simulink model "single_phase_trans_short_circ_test"  (R2024b)
settings: Solver=VariableStepAuto  StartTime=0.0  StopTime=1  RelTol=1e-3
libraries: spsRMSLib x2, spsACVoltageSourceLib x1, spsCurrentMeasurementLib x1, spsLinearTransformerLib x1, eePowerMeasurement x1, spsVoltageMeasurementLib x1, sps_lib x1
settings Model: Creator=msi-nb  LastModifiedBy=msi-nb

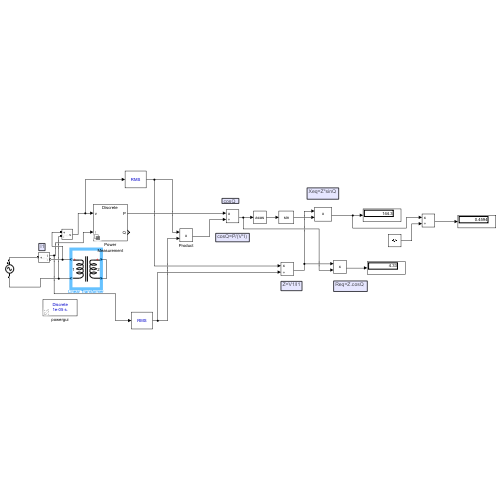
[thumbnail: Simulink's stored preview of the top-level diagram]
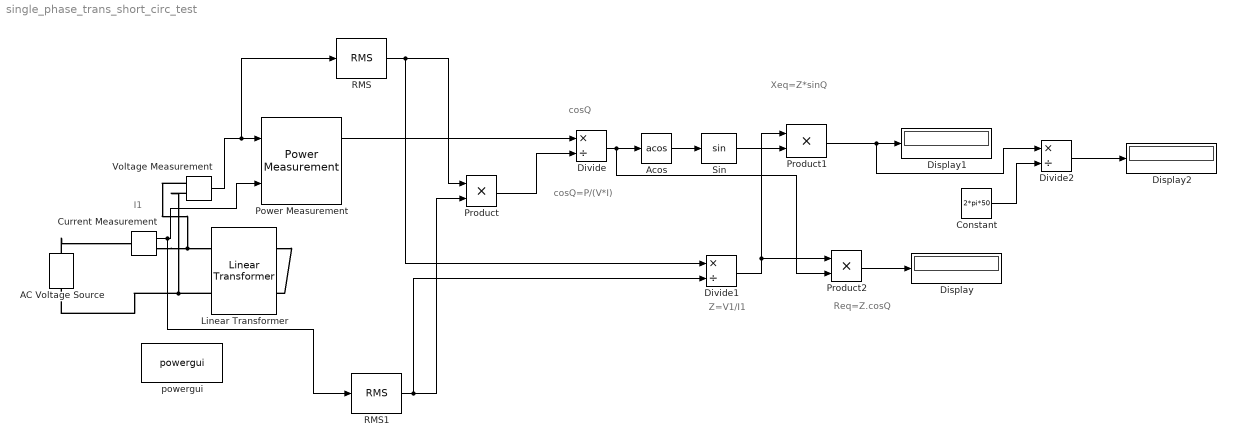
== system single_phase_trans_short_circ_test ==
  note: Xeq=Z*sinQ
  note: Req=Z.cosQ
  note: Z=V1/I1
  note: I1
  note: cosQ
  note: cosQ=P/(V*I)
  AC Voltage Source : spsACVoltageSourceLib/AC Voltage Source  Amplitude=220  Phase=0  Frequency=50  SampleTime=1e-5  Measurements=None  BusType=swing  Pref=10e3  Qref=0  Qmin=-inf  Qmax=+inf
  Acos : Trigonometry  Operator=acos
  Constant : Constant  Value=2*pi*50
  Current Measurement : spsCurrentMeasurementLib/Current Measurement  PhasorSimulation=off  OutputType=Complex  PSBequivalent=0
  Display : Display
  Display1 : Display
  Display2 : Display
  Divide : Product  Inputs=*/
  Divide1 : Product  Inputs=*/
  Divide2 : Product  Inputs=*/
  Linear Transformer : spsLinearTransformerLib/Linear Transformer  UNITS=SI  NominalPower=[ 0.5e+6 50 ]  winding1=[220 4.3218 0.45856]  winding2=[2200 0.7938 0.084225]  ThreeWindings=off  winding3=[3.15e+05 396.9 50.535]  RmLm=[1.0804e+06 2886]  Measurements=None  DataType=on
  Power Measurement : eePowerMeasurement/Power Measurement  LabelModeActiveChoice=Discrete  F=50  K=[1]  Ts=1e-5
  Product : Product
  Product1 : Product
  Product2 : Product
  RMS : spsRMSLib/RMS  TrueRMS=off  Freq=50  RMSInit=120  Ts=0
  RMS1 : spsRMSLib/RMS  TrueRMS=off  Freq=50  RMSInit=120  Ts=0
  Sin : Trigonometry
  Voltage Measurement : spsVoltageMeasurementLib/Voltage Measurement  PhasorSimulation=off  OutputType=Complex  PSBequivalent=0
  powergui : sps_lib/powergui  Priority=1  SimulationMode=Discrete  SampleTime=1e-5  frequency=60  Iterations=50  frequencyindice=50  Pbase=100e6  ErrMax=1e-4  UnitsV=kV  UnitsW=MW  buscounter=0  FunctionMessages=off  echomessages=off  EnableUseOfTLC=off  CurrentSourceSwitches=off  DisableSnubberDevices=off  DisableRonSwitches=off  DisableVfSwitches=off  DisplayEquations=off  AutomaticDiscreteSolvers=off  SolverType=Tustin/Backward Euler (TBE)  Interpol=off  ExternalGateDelay=off  methode=off  Ts=100  x0status=blocks  SPID=on  SwTol=0  HookPort=off  NonlinearTolerance=1e-4  nMaxIteration=100  ContinueOnMaxIteration=off  RestoreLinks=warning  ResistiveCurrentMeasurement=off  Frange=[0:2:500]  Ylog=off  Xlog=on  ShowGrid=off  save=off  variable=ZData  structure=0  ZoomFFT=off  StartTime=0.0  cycles=1  DisplayStyle=1  fundamental=60  FreqAxis=off  MaxFrequency=1000  frequencyindicesteady=1  RmsSteady=1  display=off
  wires:
  Current Measurement/1 -> RMS1/1, Power Measurement/2
  Power Measurement/1 -> Divide/1
  RMS/1 -> Divide1/1, Product/1
  RMS1/1 -> Divide1/2, Product/2
  Product/1 -> Divide/2
  Voltage Measurement/1 -> RMS/1, Power Measurement/1
  Divide/1 -> Product2/2, Acos/1
  Divide1/1 -> Product2/1, Product1/1
  Sin/1 -> Product1/2
  Acos/1 -> Sin/1
  Product2/1 -> Display/1
  Product1/1 -> Divide2/1, Display1/1
  Divide2/1 -> Display2/1
  Constant/1 -> Divide2/2
  connections:
  AC Voltage Source/RConn1 -- Current Measurement/LConn1
  Current Measurement/RConn1 -- Voltage Measurement/LConn1 -- Linear Transformer/LConn1
  Linear Transformer/LConn2 -- Voltage Measurement/LConn2 -- AC Voltage Source/LConn1
  Linear Transformer/RConn1 -- Linear Transformer/RConn2
